simulink model "k1visitmxt"  (Simulink 8.6)
settings: Solver=ode45  StartTime=0.0  StopTime=10.0  RelTol=1e-3
libraries: cdsIPCx x27, cdsCDI64 x4, cdsCDO64 x4, BIO_CD_ENCODE_MASTER x4, BIO_CD_DECODE_MASTER x4, CHK_DIO x4, cdsFilt x3, cdsAdcx0 x1, cdsCDO32 x1, dac x1, TYPEA_MASTER x1, BO_TYPEA_MASTER x1
settings Model: Creator=controls  LastModifiedBy=controls
settings DataIOCC: SignalLoggingSaveFormat=Dataset
settings OptimizationCC: ExpressionDepthLimit=128
settings DebuggingCC: UnderspecifiedInitializationDetection=Simplified  MergeDetectMultiDrivingBlocksExec=error  SolverPrmCheckMsg=none  FcnCallInpInsideContextMsg=EnableAllAsError  StateNameClashWarn=none
settings GRTTargetCC: CombineOutputUpdateFcns=on  GRTInterface=off

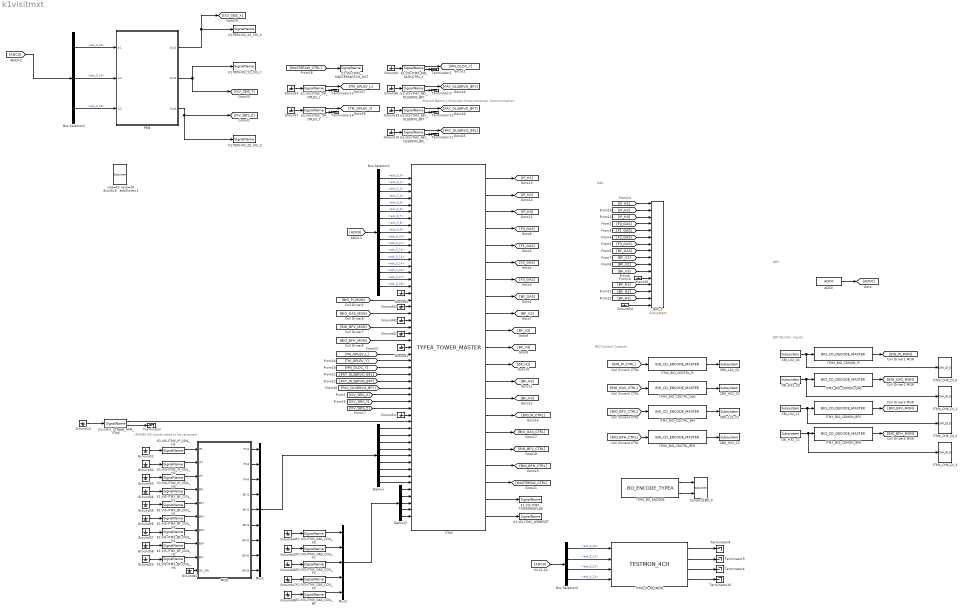
== system k1visitmxt ==
  note: BIO Monitor Inputs
  note: BIO Control Outputs
  note: DAC
  note: ADC
  note: Shared Memory Channels
      | Inner-computer Communication
  note: [FIXME] IPC blocks need to be renamed
  ADC0 : cdsAdcx0/ADC0  Tag=cdsAdc  Description=|
      | type-GSC_16AI64SSA
      | card_num=0
      settings: AttributesFormatString=%<Description>\n%<Tag>
  Bus Selector1 : BusSelector  OutputSignals=adc_0_0,adc_0_1,adc_0_2,adc_0_4,adc_0_5,adc_0_6,adc_0_7,adc_0_8,adc_0_9,adc_0_10,adc_0_11,adc_0_12,adc_0_13,adc_0_14,adc_0_16,adc_0_17,adc_0_18
  Bus Selector2 : BusSelector  OutputSignals=adc_0_24,adc_0_25,adc_0_26
  Bus Selector3 : BusSelector  OutputSignals=adc_0_20,adc_0_21,adc_0_22,adc_0_23
  CBI_H32_C0 : cdsCDI64/Subsystem  Tag=cdsCDI64  Description=card_num=1
      settings: AttributesFormatString=%<Tag>\n%<Description>
  CBI_H32_C1 : cdsCDI64/Subsystem  Tag=cdsCDI64  Description=card_num=3
      settings: AttributesFormatString=%<Tag>\n%<Description>
  CBI_L32_C0 : cdsCDI64/Subsystem  Tag=cdsCDI64  Description=card_num=0
      settings: AttributesFormatString=%<Tag>\n%<Description>
  CBI_L32_C1 : cdsCDI64/Subsystem  Tag=cdsCDI64  Description=card_num=2
      settings: AttributesFormatString=%<Tag>\n%<Description>
  CBO_H32_C0 : cdsCDO64/Subsystem  Tag=cdsCDO64  Description=card_num=1
      settings: AttributesFormatString=%<Tag>\n%<Description>
  CBO_H32_C1 : cdsCDO64/Subsystem  Tag=cdsCDO64  Description=card_num=3
      settings: AttributesFormatString=%<Tag>\n%<Description>
  CBO_L32_C0 : cdsCDO64/Subsystem  Tag=cdsCDO64  Description=card_num=0
      settings: AttributesFormatString=%<Tag>\n%<Description>
  CBO_L32_C1 : cdsCDO64/Subsystem  Tag=cdsCDO64  Description=card_num=2
      settings: AttributesFormatString=%<Tag>\n%<Description>
  Contec32BO_0 : cdsCDO32/Subsystem  Tag=cdsCDO32  Description=Contec32 bit binary output module driver
      settings: AttributesFormatString=%<Tag>
  DAC_0 : dac/Subsystem  Description=|
      | type=GSC_16AO16,
      | card_num=0
      settings: AttributesFormatString=%<Description>
  Demux : Demux  Outputs=9
  Demux2 : Demux  Outputs=5
  Ground{1..7,10..11,13..14,24,31..48} (30 alike) : Ground
  ITMX : TYPEA_MASTER/TYPEA_TOWER_MASTER
  ITMX_BIO_CDCTRL_BFH : BIO_CD_ENCODE_MASTER/BIO_CD_ENCODE_MASTER
  ITMX_BIO_CDCTRL_BFV : BIO_CD_ENCODE_MASTER/BIO_CD_ENCODE_MASTER
  ITMX_BIO_CDCTRL_GAS : BIO_CD_ENCODE_MASTER/BIO_CD_ENCODE_MASTER
  ITMX_BIO_CDCTRL_PI : BIO_CD_ENCODE_MASTER/BIO_CD_ENCODE_MASTER
  ITMX_BIO_CDMON_BFH : BIO_CD_DECODE_MASTER/BIO_CD_DECODE_MASTER
  ITMX_BIO_CDMON_BFV : BIO_CD_DECODE_MASTER/BIO_CD_DECODE_MASTER
  ITMX_BIO_CDMON_GAS : BIO_CD_DECODE_MASTER/BIO_CD_DECODE_MASTER
  ITMX_BIO_CDMON_PI : BIO_CD_DECODE_MASTER/BIO_CD_DECODE_MASTER
  ITMX_BO_ENCODE : BO_TYPEA_MASTER/BO_ENCODE_TYPEA
  ITMX_CHK_DI_{0..3} (4 alike) : CHK_DIO/CHK_DI_0
  ITMX_IP_ACCMON : TESTMON_4CH_MASTER/TESTMON_4CH
  K1:GIF-X_STRAIN_RFM_ITMX : cdsIPCx/SignalName  Tag=cdsIPCx_RFM  Description=card=0
      settings: AttributesFormatString=%<Description>\n%<Tag>
  K1:PEM-IXV_X2_VIS_X : cdsIPCx/SignalName  Tag=cdsIPCx_RFM  Description=card=0
      settings: AttributesFormatString=%<Description>\n%<Tag>
  K1:PEM-IXV_Y2_VIS_Y : cdsIPCx/SignalName  Tag=cdsIPCx_RFM  Description=card=0
      settings: AttributesFormatString=%<Description>\n%<Tag>
  K1:PEM-IXV_Z2_VIS_Z : cdsIPCx/SignalName  Tag=cdsIPCx_RFM  Description=card=0
      settings: AttributesFormatString=%<Description>\n%<Tag>
  K1:VIS-ITMX_BF_COIL_H1 : cdsIPCx/SignalName  Tag=cdsIPCx_SHMEM  Description=Inter-Process Communication via Shared memory.
      settings: AttributesFormatString=%<Tag>
  K1:VIS-ITMX_BF_COIL_H2 : cdsIPCx/SignalName  Tag=cdsIPCx_SHMEM  Description=Inter-Process Communication via Shared memory.
      settings: AttributesFormatString=%<Tag>
  K1:VIS-ITMX_BF_COIL_H3 : cdsIPCx/SignalName  Tag=cdsIPCx_SHMEM  Description=Inter-Process Communication via Shared memory.
      settings: AttributesFormatString=%<Tag>
  K1:VIS-ITMX_BF_COIL_V1 : cdsIPCx/SignalName  Tag=cdsIPCx_SHMEM  Description=Inter-Process Communication via Shared memory.
      settings: AttributesFormatString=%<Tag>
  K1:VIS-ITMX_BF_COIL_V2 : cdsIPCx/SignalName  Tag=cdsIPCx_SHMEM  Description=Inter-Process Communication via Shared memory.
      settings: AttributesFormatString=%<Tag>
  K1:VIS-ITMX_BF_COIL_V3 : cdsIPCx/SignalName  Tag=cdsIPCx_SHMEM  Description=Inter-Process Communication via Shared memory.
      settings: AttributesFormatString=%<Tag>
  K1:VIS-ITMX_GAS_COIL_BF : cdsIPCx/SignalName  Tag=cdsIPCx_SHMEM  Description=Inter-Process Communication via Shared memory.
      settings: AttributesFormatString=%<Tag>
  K1:VIS-ITMX_GAS_COIL_F{0..3} (4 alike) : cdsIPCx/SignalName  Tag=cdsIPCx_SHMEM  Description=Inter-Process Communication via Shared memory.
      settings: AttributesFormatString=%<Tag>
  K1:VIS-ITMX_IP_COIL_H1 : cdsIPCx/SignalName  Tag=cdsIPCx_SHMEM  Description=Inter-Process Communication via Shared memory.
      settings: AttributesFormatString=%<Tag>
  K1:VIS-ITMX_IP_COIL_H2 : cdsIPCx/SignalName  Tag=cdsIPCx_SHMEM  Description=Inter-Process Communication via Shared memory.
      settings: AttributesFormatString=%<Tag>
  K1:VIS-ITMX_IP_COIL_H3 : cdsIPCx/SignalName  Tag=cdsIPCx_SHMEM  Description=Inter-Process Communication via Shared memory.
      settings: AttributesFormatString=%<Tag>
  K1:VIS-ITMX_MASTERSWITCH_OUT : cdsIPCx/SignalName  Tag=cdsIPCx_SHMEM  Description=Inter-Process Communication via Shared memory.
      settings: AttributesFormatString=%<Tag>
  K1:VIS-ITMX_MN_OLDCCTRL_Y : cdsIPCx/SignalName  Tag=cdsIPCx_SHMEM  Description=Inter-Process Communication via Shared memory.
      settings: AttributesFormatString=%<Tag>
  K1:VIS-ITMX_PAY_OLSERVO_BFL : cdsIPCx/SignalName  Tag=cdsIPCx_SHMEM  Description=Inter-Process Communication via Shared memory.
      settings: AttributesFormatString=%<Tag>
  K1:VIS-ITMX_PAY_OLSERVO_BFT : cdsIPCx/SignalName  Tag=cdsIPCx_SHMEM  Description=Inter-Process Communication via Shared memory.
      settings: AttributesFormatString=%<Tag>
  K1:VIS-ITMX_PAY_OLSERVO_BFY : cdsIPCx/SignalName  Tag=cdsIPCx_SHMEM  Description=Inter-Process Communication via Shared memory.
      settings: AttributesFormatString=%<Tag>
  K1:VIS-ITMX_TM_OPLEV_L : cdsIPCx/SignalName  Tag=cdsIPCx_SHMEM  Description=Inter-Process Communication via Shared memory.
      settings: AttributesFormatString=%<Tag>
  K1:VIS-ITMX_TM_OPLEV_Y : cdsIPCx/SignalName  Tag=cdsIPCx_SHMEM  Description=Inter-Process Communication via Shared memory.
      settings: AttributesFormatString=%<Tag>
  K1:VIS-ITMX_TOWERWDFLAG : cdsIPCx/SignalName  Tag=cdsIPCx_SHMEM  Description=Inter-Process Communication via Shared memory.
      settings: AttributesFormatString=%<Tag>
  K1:VIS-ITMX_WDRESET : cdsIPCx/SignalName  Tag=cdsIPCx_SHMEM  Description=Inter-Process Communication via Shared memory.
      settings: AttributesFormatString=%<Tag>
  MOD : Subsystem  Tag=top_names
  Mux1 : Mux  Inputs=9
  Mux2 : Mux  Inputs=5
  PEM : Subsystem  Tag=top_names
      settings: AttributesFormatString=%<Tag>
  Terminator{,1,3..4,8..14} (11 alike) : Terminator
  site=K1 rate=2K dcuid=66 host=k1ix1 specific_cpu=3 adcSlave=1 : cdsParameters/Subsystem  Tag=cdsParameters  Description=|
      | Purpose:                                                                                                                                                                                                                                
      | Provide system parameters to the FE code generator to properly configure the generated EPICS names, rep rate of the FE controller, and the Data Acquisition node ID for proper storage of data from this FE controller.                 
      |                                                                                                                                                                                                                                         
      | Useage:                                                                                                                                                                                                                                 
      | The part NAME field is used to identify the FE parameters. It must be of the form:                                                                                                                                                      
      | site=                                                                                                                                                                                                                                   
      | rate=                                                                                                                                                                                                                                   
      | dcuid=                                                                                                                                                                                                                                  
      |                                                                                                                                                                                                                                         
      | Where:                                                                                                                                                                                                                                  
      | site= argument may be H1, H2, L1, M1, G1, either as a single argument or multiple, for example site=H1,H2. These are the only names allowed. These will become the first two characters of all EPICS and signal names (for example G1:).
      |                                                                                                                                                                                                                                         
      | rate= may be 2K, 16K, 32K, or 64K                                                                                                                                                                                                       
      |                                                                                                                                                                                                                                         
      | dcuid= is site specific ie it must be unique at each site.
      settings: AttributesFormatString=%<Tag>
  wires:
  ADC0/1 -> [ADC0]
  ITMX/4 -> [F0_GAS]
  ITMX/5 -> [F1_GAS]
  ITMX/8 -> [BF_GAS]
  ITMX/7 -> [F3_GAS]
  ITMX/6 -> [F2_GAS]
  ITMX/9 -> [BF_V1]
  ITMX/10 -> [BF_V2]
  ITMX/11 -> [BF_V3]
  ITMX/12 -> [BF_H1]
  ITMX/13 -> [BF_H2]
  ITMX/14 -> [BF_H3]
  [BF_H2] -> DAC_0/14
  [BF_V3] -> DAC_0/11
  [BF_H3] -> DAC_0/15
  [BF_V1] -> DAC_0/9
  [BF_H1] -> DAC_0/13
  [BF_V2] -> DAC_0/10
  ITMX/1 -> [IP_H1]
  ITMX/2 -> [IP_H2]
  ITMX/3 -> [IP_H3]
  CBI_H32_C0/1 -> ITMX_CHK_DI_1/1, ITMX_BIO_CDMON_GAS/1
  CBI_L32_C1/1 -> ITMX_CHK_DI_2/1, ITMX_BIO_CDMON_BFV/1
  CBI_L32_C0/1 -> ITMX_CHK_DI_0/1, ITMX_BIO_CDMON_PI/1
  CBI_H32_C1/1 -> ITMX_CHK_DI_3/1, ITMX_BIO_CDMON_BFH/1
  ITMX_BIO_CDCTRL_BFH/1 -> CBO_H32_C1/1
  ITMX_BIO_CDCTRL_PI/1 -> CBO_L32_C0/1
  ITMX_BIO_CDCTRL_GAS/1 -> CBO_H32_C0/1
  ITMX_BIO_CDCTRL_BFV/1 -> CBO_L32_C1/1
  [BIO_PI_CTRL] -> ITMX_BIO_CDCTRL_PI/1
  [BIO_GAS_CTRL] -> ITMX_BIO_CDCTRL_GAS/1
  [BIO_BFV_CTRL] -> ITMX_BIO_CDCTRL_BFV/1
  ITMX_BIO_CDMON_PI/1 -> [BIO_PI_MON]
  ITMX_BIO_CDMON_GAS/1 -> [BIO_GAS_MON]
  ITMX_BIO_CDMON_BFH/1 -> [BIO_BFH_MON]
  ITMX_BIO_CDMON_BFV/1 -> [BIO_BFV_MON]
  [BIO_BFH_CTRL] -> ITMX_BIO_CDCTRL_BFH/1
  [IP_H1] -> DAC_0/1
  [IP_H2] -> DAC_0/2
  [IP_H3] -> DAC_0/3
  [F0_GAS] -> DAC_0/4
  [F1_GAS] -> DAC_0/5
  [F2_GAS] -> DAC_0/6
  [F3_GAS] -> DAC_0/7
  [BF_GAS] -> DAC_0/8
  [ADC0] -> Bus Selector3/1
  Bus Selector3/2 -> ITMX_IP_ACCMON/2  "<adc_0_21>"
  Bus Selector3/1 -> ITMX_IP_ACCMON/1  "<adc_0_20>"
  Bus Selector3/3 -> ITMX_IP_ACCMON/3  "<adc_0_22>"
  Bus Selector3/4 -> ITMX_IP_ACCMON/4  "<adc_0_23>"
  ITMX_IP_ACCMON/3 -> Terminator4/1
  ITMX_IP_ACCMON/4 -> Terminator10/1
  ITMX_IP_ACCMON/1 -> Terminator8/1
  ITMX_IP_ACCMON/2 -> Terminator9/1
  Ground5/1 -> DAC_0/12
  Ground24/1 -> DAC_0/16
  ITMX/15 -> [BIO_PI_CTRL]
  ITMX/16 -> [BIO_GAS_CTRL]
  ITMX/17 -> [BIO_BFV_CTRL]
  ITMX/18 -> [BIO_BFH_CTRL]
  ITMX_BO_ENCODE/1 -> Contec32BO_0/1
  ITMX_BO_ENCODE/2 -> Contec32BO_0/2
  [ADC0] -> Bus Selector1/1
  Bus Selector1/1 -> ITMX/1  "<adc_0_0>"
  Bus Selector1/2 -> ITMX/2  "<adc_0_1>"
  Bus Selector1/3 -> ITMX/3  "<adc_0_2>"
  Bus Selector1/4 -> ITMX/4  "<adc_0_4>"
  Bus Selector1/5 -> ITMX/5  "<adc_0_5>"
  Bus Selector1/6 -> ITMX/6  "<adc_0_6>"
  Bus Selector1/7 -> ITMX/7  "<adc_0_7>"
  Bus Selector1/8 -> ITMX/8  "<adc_0_8>"
  Bus Selector1/9 -> ITMX/9  "<adc_0_9>"
  Bus Selector1/10 -> ITMX/10  "<adc_0_10>"
  Bus Selector1/11 -> ITMX/11  "<adc_0_11>"
  Bus Selector1/12 -> ITMX/12  "<adc_0_12>"
  Bus Selector1/13 -> ITMX/13  "<adc_0_13>"
  Bus Selector1/14 -> ITMX/14  "<adc_0_14>"
  Bus Selector1/15 -> ITMX/15  "<adc_0_16>"
  Bus Selector1/16 -> ITMX/16  "<adc_0_17>"
  Bus Selector1/17 -> ITMX/17  "<adc_0_18>"
  [BIO_PI_MON] -> ITMX/19
  [BIO_GAS_MON] -> ITMX/21
  [BIO_BFV_MON] -> ITMX/23
  [BIO_BFH_MON] -> ITMX/25
  Ground43/1 -> ITMX/20
  Ground41/1 -> ITMX/22
  Ground42/1 -> ITMX/24
  Ground2/1 -> ITMX/18
  K1:VIS-ITMX_PAY_OLSERVO_BFY/2 -> Terminator3/1
  K1:VIS-ITMX_MN_OLDCCTRL_Y/2 -> Terminator1/1
  Ground4/1 -> K1:VIS-ITMX_MN_OLDCCTRL_Y/1
  Ground6/1 -> K1:VIS-ITMX_PAY_OLSERVO_BFY/1
  K1:VIS-ITMX_MN_OLDCCTRL_Y/1 -> [MN_OLDC_Y]
  K1:VIS-ITMX_PAY_OLSERVO_BFY/1 -> [PAY_OLSERVO_BFY]
  K1:VIS-ITMX_PAY_OLSERVO_BFL/2 -> Terminator11/1
  Ground10/1 -> K1:VIS-ITMX_PAY_OLSERVO_BFL/1
  K1:VIS-ITMX_PAY_OLSERVO_BFL/1 -> [PAY_OLSERVO_BFL]
  K1:VIS-ITMX_PAY_OLSERVO_BFT/2 -> Terminator12/1
  Ground13/1 -> K1:VIS-ITMX_PAY_OLSERVO_BFT/1
  K1:VIS-ITMX_PAY_OLSERVO_BFT/1 -> [PAY_OLSERVO_BFT]
  K1:VIS-ITMX_TM_OPLEV_L/2 -> Terminator13/1
  Ground3/1 -> K1:VIS-ITMX_TM_OPLEV_L/1
  K1:VIS-ITMX_TM_OPLEV_L/1 -> [TM_OPLEV_L]
  K1:VIS-ITMX_TM_OPLEV_Y/2 -> Terminator14/1
  Ground7/1 -> K1:VIS-ITMX_TM_OPLEV_Y/1
  K1:VIS-ITMX_TM_OPLEV_Y/1 -> [TM_OPLEV_Y]
  Ground14/1 -> K1:GIF-X_STRAIN_RFM_ITMX/1
  K1:GIF-X_STRAIN_RFM_ITMX/2 -> Terminator/1
  ITMX/19 -> [MASTERSW_CTRL]
  ITMX/20 -> K1:VIS-ITMX_TOWERWDFLAG/1
  ITMX/21 -> K1:VIS-ITMX_WDRESET/1
  [MASTERSW_CTRL] -> K1:VIS-ITMX_MASTERSWITCH_OUT/1
  Ground11/1 -> ITMX/36
  [IXV_SEIS_Z] -> ITMX/35
  [IXV_SEIS_Y] -> ITMX/34
  [IXV_SEIS_X] -> ITMX/33
  [PAY_OLSERVO_BFY] -> ITMX/32
  [PAY_OLSERVO_BFT] -> ITMX/31
  [PAY_OLSERVO_BFL] -> ITMX/30
  [MN_OLDC_Y] -> ITMX/29
  [TM_OPLEV_Y] -> ITMX/28
  [TM_OPLEV_L] -> ITMX/27
  Ground1/1 -> ITMX/26
  K1:GIF-X_STRAIN_RFM_ITMX/1 -> ITMX/37
  Mux1/1 -> Demux/1
  Demux/1 -> ITMX/38
  Demux/2 -> ITMX/39
  Demux/3 -> ITMX/40
  Demux/4 -> ITMX/41
  Demux/5 -> ITMX/42
  Demux/6 -> ITMX/43
  Demux/7 -> ITMX/44
  Demux/8 -> ITMX/45
  Demux/9 -> ITMX/46
  [ADC0] -> Bus Selector2/1
  Bus Selector2/1 -> PEM/1(In1)  "<adc_0_24>"
  Bus Selector2/2 -> PEM/2(In2)  "<adc_0_25>"
  Bus Selector2/3 -> PEM/3(In3)  "<adc_0_26>"
  PEM/1(Out1) -> [IXV_SEIS_X], K1:PEM-IXV_X2_VIS_X/1
  PEM/2(Out2) -> [IXV_SEIS_Y], K1:PEM-IXV_Y2_VIS_Y/1
  PEM/3(Out3) -> [IXV_SEIS_Z], K1:PEM-IXV_Z2_VIS_Z/1
  Ground31/1 -> K1:VIS-ITMX_IP_COIL_H1/1
  Ground32/1 -> K1:VIS-ITMX_IP_COIL_H2/1
  Ground33/1 -> K1:VIS-ITMX_IP_COIL_H3/1
  Ground34/1 -> K1:VIS-ITMX_BF_COIL_V1/1
  Ground35/1 -> K1:VIS-ITMX_BF_COIL_V2/1
  Ground36/1 -> K1:VIS-ITMX_BF_COIL_V3/1
  Ground37/1 -> K1:VIS-ITMX_BF_COIL_H1/1
  Ground38/1 -> K1:VIS-ITMX_BF_COIL_H2/1
  Ground39/1 -> K1:VIS-ITMX_BF_COIL_H3/1
  K1:VIS-ITMX_IP_COIL_H1/1 -> MOD/1(IPL)
  K1:VIS-ITMX_IP_COIL_H2/1 -> MOD/2(IPT)
  K1:VIS-ITMX_IP_COIL_H3/1 -> MOD/3(IPY)
  K1:VIS-ITMX_BF_COIL_V1/1 -> MOD/4(BFL)
  K1:VIS-ITMX_BF_COIL_V2/1 -> MOD/5(BFT)
  K1:VIS-ITMX_BF_COIL_V3/1 -> MOD/6(BFV)
  K1:VIS-ITMX_BF_COIL_H1/1 -> MOD/7(BFR)
  K1:VIS-ITMX_BF_COIL_H2/1 -> MOD/8(BFP)
  K1:VIS-ITMX_BF_COIL_H3/1 -> MOD/9(BFY)
  MOD/1(IPH1) -> Mux1/1
  MOD/2(IPH2) -> Mux1/2
  MOD/3(IPH3) -> Mux1/3
  MOD/4(BFV1) -> Mux1/4
  MOD/5(BFV2) -> Mux1/5
  MOD/6(BFV3) -> Mux1/6
  MOD/7(BFH1) -> Mux1/7
  MOD/8(BFH2) -> Mux1/8
  MOD/9(BFH3) -> Mux1/9
  Ground40/1 -> MOD/10(ISC_MN)
  K1:VIS-ITMX_GAS_COIL_F0/1 -> Mux2/1
  K1:VIS-ITMX_GAS_COIL_F1/1 -> Mux2/2
  K1:VIS-ITMX_GAS_COIL_F2/1 -> Mux2/3
  K1:VIS-ITMX_GAS_COIL_F3/1 -> Mux2/4
  K1:VIS-ITMX_GAS_COIL_BF/1 -> Mux2/5
  Ground44/1 -> K1:VIS-ITMX_GAS_COIL_F0/1
  Ground45/1 -> K1:VIS-ITMX_GAS_COIL_F1/1
  Ground46/1 -> K1:VIS-ITMX_GAS_COIL_F2/1
  Ground47/1 -> K1:VIS-ITMX_GAS_COIL_F3/1
  Ground48/1 -> K1:VIS-ITMX_GAS_COIL_BF/1
  Mux2/1 -> Demux2/1
  Demux2/1 -> ITMX/47
  Demux2/2 -> ITMX/48
  Demux2/3 -> ITMX/49
  Demux2/4 -> ITMX/50
  Demux2/5 -> ITMX/51

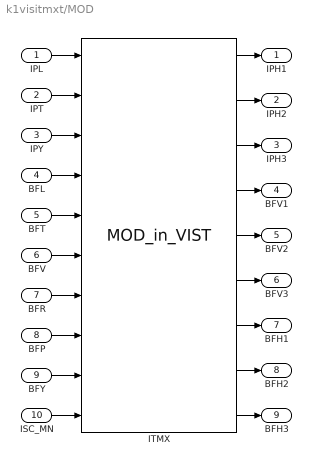
== system k1visitmxt/MOD ==
  IPL : Inport
  IPT : Inport  Port=2
  IPY : Inport  Port=3
  BFL : Inport  Port=4
  BFT : Inport  Port=5
  BFV : Inport  Port=6
  BFR : Inport  Port=7
  BFP : Inport  Port=8
  BFY : Inport  Port=9
  ISC_MN : Inport  Port=10
  ITMX : VIS_LIB/MODAL/MOD_in_VIST  Tag=top_names
  IPH1 : Outport
  IPH2 : Outport  Port=2
  IPH3 : Outport  Port=3
  BFV1 : Outport  Port=4
  BFV2 : Outport  Port=5
  BFV3 : Outport  Port=6
  BFH1 : Outport  Port=7
  BFH2 : Outport  Port=8
  BFH3 : Outport  Port=9
  wires:
  IPL/1 -> ITMX/1
  IPT/1 -> ITMX/2
  IPY/1 -> ITMX/3
  BFL/1 -> ITMX/4
  BFT/1 -> ITMX/5
  BFV/1 -> ITMX/6
  BFR/1 -> ITMX/7
  BFP/1 -> ITMX/8
  BFY/1 -> ITMX/9
  ITMX/1 -> IPH1/1
  ITMX/2 -> IPH2/1
  ITMX/3 -> IPH3/1
  ITMX/4 -> BFV1/1
  ITMX/5 -> BFV2/1
  ITMX/6 -> BFV3/1
  ITMX/7 -> BFH1/1
  ITMX/8 -> BFH2/1
  ITMX/9 -> BFH3/1
  ISC_MN/1 -> ITMX/10

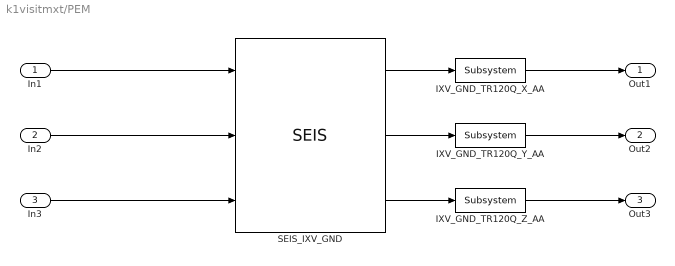
== system k1visitmxt/PEM ==
  In1 : Inport
  In2 : Inport  Port=2
  In3 : Inport  Port=3
  IXV_GND_TR120Q_X_AA : cdsFilt/Subsystem  Tag=cdsFilt  Description=|
      | Purpose:                                                                                                                                                                                                                                  
      | Standard CDS IIR filter module.                                                                                                                                                                                                           
      |                                                                                                                                                                                                                                           
      | Operation:                                                                                                                                                                                                                                
      | Consists of 10 second order section IIR filters, plus a ramped gain stage. In FE code, also provides pre-defined test points and excitation channel inputs. The filter coefficients are defined in the LIGO system using the 'foton' tool.
      |                                                                                                                                                                                                                                           
      | Usage:                                                                                                                                                                                                                                    
      | Name the part with the desired filter module name.
      settings: AttributesFormatString=%<Tag>
  IXV_GND_TR120Q_Y_AA : cdsFilt/Subsystem  Tag=cdsFilt  Description=|
      | Purpose:                                                                                                                                                                                                                                  
      | Standard CDS IIR filter module.                                                                                                                                                                                                           
      |                                                                                                                                                                                                                                           
      | Operation:                                                                                                                                                                                                                                
      | Consists of 10 second order section IIR filters, plus a ramped gain stage. In FE code, also provides pre-defined test points and excitation channel inputs. The filter coefficients are defined in the LIGO system using the 'foton' tool.
      |                                                                                                                                                                                                                                           
      | Usage:                                                                                                                                                                                                                                    
      | Name the part with the desired filter module name.
      settings: AttributesFormatString=%<Tag>
  IXV_GND_TR120Q_Z_AA : cdsFilt/Subsystem  Tag=cdsFilt  Description=|
      | Purpose:                                                                                                                                                                                                                                  
      | Standard CDS IIR filter module.                                                                                                                                                                                                           
      |                                                                                                                                                                                                                                           
      | Operation:                                                                                                                                                                                                                                
      | Consists of 10 second order section IIR filters, plus a ramped gain stage. In FE code, also provides pre-defined test points and excitation channel inputs. The filter coefficients are defined in the LIGO system using the 'foton' tool.
      |                                                                                                                                                                                                                                           
      | Usage:                                                                                                                                                                                                                                    
      | Name the part with the desired filter module name.
      settings: AttributesFormatString=%<Tag>
  SEIS_IXV_GND : seis/SEIS
  Out1 : Outport
  Out2 : Outport  Port=2
  Out3 : Outport  Port=3
  wires:
  IXV_GND_TR120Q_X_AA/1 -> Out1/1
  IXV_GND_TR120Q_Y_AA/1 -> Out2/1
  IXV_GND_TR120Q_Z_AA/1 -> Out3/1
  SEIS_IXV_GND/2 -> IXV_GND_TR120Q_Y_AA/1
  In1/1 -> SEIS_IXV_GND/1
  In2/1 -> SEIS_IXV_GND/2
  In3/1 -> SEIS_IXV_GND/3
  SEIS_IXV_GND/1 -> IXV_GND_TR120Q_X_AA/1
  SEIS_IXV_GND/3 -> IXV_GND_TR120Q_Z_AA/1
